simulink model "hapticsSimBlk_pd"  (Simulink 6.5)
settings: Solver=FixedStepDiscrete  StartTime=0.0  StopTime=20  FixedStep=0.00001  RelTol=1e-3
libraries: simulink x1, RT x1
settings Model: Creator=Mengchen  LastModifiedBy=Sara
settings DebuggingCC: AlgebraicLoopMsg=error  SignalResolutionControl=UseLocalSettings
settings HardwareCC: TargetEndianess=LittleEndian  TargetHWDeviceType=MATLAB Host
settings RTWCC: ProcessScript=grt_make_rtw_hook  CustomHeaderCode="#include \"haptics.h\""  CustomInclude="\"C:\\Program Files\\novint\\HDAL_SDK_1.1.0_Beta\\include\""  TargetLang=C++
settings GRTTargetCC: TargetFcnLib=ansi_tfl_table_tmw.mat

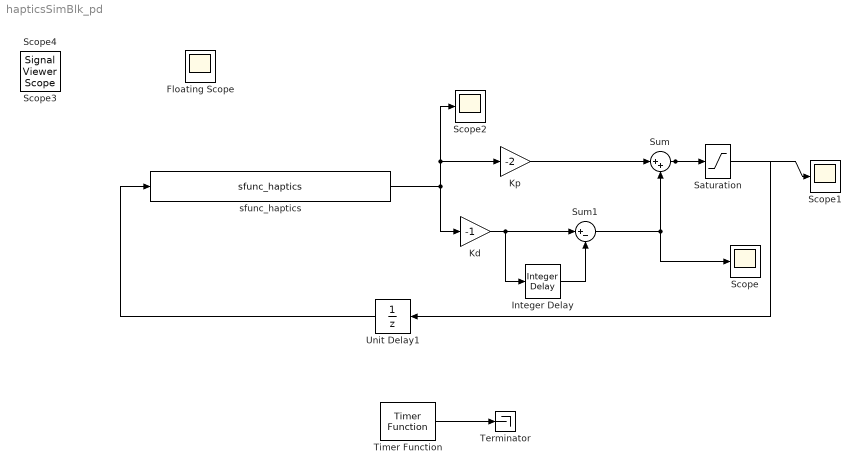
== system hapticsSimBlk_pd ==
  Integer Delay : simulink/Discrete/Integer Delay  vinit=0.0  samptime=-1  NumDelays=2
  Kd : Gain  Gain=-1
  Kp : Gain  Gain=-2
  Saturation : Saturate  UpperLimit=200  LowerLimit=-200
  Scope : Scope
      settings: YMin=-0.9  YMax=0.6
  Scope1 : Scope
  Scope2 : Scope
      settings: YMin=-1.2  YMax=1  SaveName=ScopeData2
  Sum : Sum  Inputs=|++
  Sum1 : Sum  Inputs=|+-
  Terminator : Terminator
  Timer Function : RT/Timer Function  step1=1  priority1=HIGH  ThPriority1=TIME CRITICAL
  Unit Delay1 : UnitDelay  Orientation=left  SampleTime=-1
  sfunc_haptics : S-Function  FunctionName=sfunc_haptics  mask(Legacy Function){SFunctionSpec=void falconPlant(double u1[3], double y1[3]), ShowSpec=on}
      mask prompts: ShowSpec "Display function specification"
      mask help:
      | This block allows the user to call the following C function(s) in Simulink:
      |
      | StartFcn: createHaptics()
      |
      | OutputFcn: void falconPlant(double u1[3], double y1[3])
      |
      | TerminateFcn: deleteHaptics()
      mask CallbackString:
      | |if strcmp(get_param(gcbh, 'ShowSpec'), 'on')
      |   set_param(gcbh, 'MaskDisplay', sprintf('fprintf(''%s'');', get_param(gcbh, 'SFunctionSpec')));
      | else
      |   set_param(gcbh, 'MaskDisplay', sprintf('fprintf(''%s'');', get_param(gcbh, 'FunctionName')));
      | end
      mask Display: fprintf('void falconPlant(double u1[3], double y1[3])');
  Floating Scope : Scope
      settings: Floating=on  SaveName=ScopeData3
  Scope3 : SignalViewerScope  IOType=viewer  RefreshTime=0.035000
  Scope4 : SignalViewerScope  IOType=viewer  RefreshTime=0.035000
  wires:
  sfunc_haptics/1 -> Kd/1, Kp/1, Scope2/1
  Kp/1 -> Sum/1
  Sum/1 -> Saturation/1
  Saturation/1 -> Scope1/1, Unit Delay1/1
  Kd/1 -> Sum1/1, Integer Delay/1
  Unit Delay1/1 -> sfunc_haptics/1
  Sum1/1 -> Sum/2, Scope/1
  Integer Delay/1 -> Sum1/2
  Timer Function/1 -> Terminator/1
